simulink library "gyroscopes"  (R2023b)
settings: Solver=VariableStepAuto  StartTime=0.0  StopTime=10.0  RelTol=1e-3
undefined symbols (not defined in the file): gyr_bias, gyr_dynamic, gyr_freq, gyr_noise, gyr_non_orthogonality
libraries: simulink x1
settings Model: Creator=robin  LastModifiedBy=robin

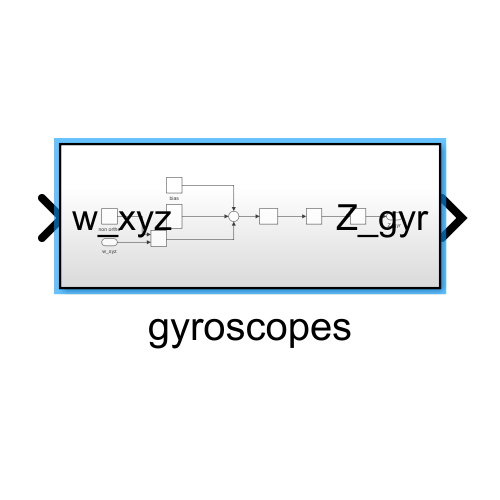
[thumbnail: Simulink's stored preview of the top-level diagram]
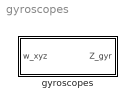
== system gyroscopes ==
  gyroscopes : Subsystem

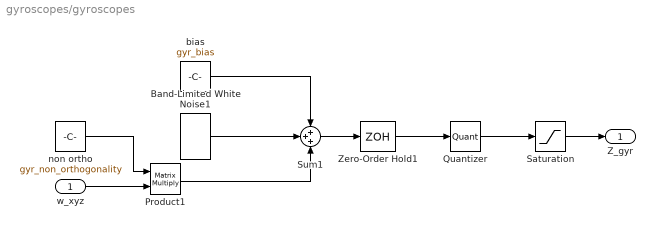
== system gyroscopes/gyroscopes ==
  w_xyz : Inport
  Band-Limited White Noise1 : simulink/Sources/Band-Limited White Noise  Cov=[2*(2*pi*gyr_noise/gyr_freq)^2 2*(2*pi*gyr_noise/gyr_freq)^2 2*(2*pi*gyr_noise/gyr_freq)^2]  Ts=1/gyr_freq  seed=[randi(1000) randi(1000) randi(1000)]  VectorParams1D=off
  Product1 : Product  Multiplication=Matrix(*)
  Quantizer : Quantizer  QuantizationInterval=gyr_res
  Saturation : Saturate  UpperLimit=gyr_dynamic  LowerLimit=-gyr_dynamic
  Sum1 : Sum  Inputs=+++
  Zero-Order Hold1 : ZeroOrderHold  SampleTime=1/gyr_freq
  bias : Constant  Value=gyr_bias
  non ortho : Constant  Value=gyr_non_orthogonality
  Z_gyr : Outport
  wires:
  non ortho/1 -> Product1/1
  Band-Limited White Noise1/1 -> Sum1/2
  bias/1 -> Sum1/1
  w_xyz/1 -> Product1/2
  Product1/1 -> Sum1/3
  Saturation/1 -> Z_gyr/1
  Zero-Order Hold1/1 -> Quantizer/1
  Sum1/1 -> Zero-Order Hold1/1
  Quantizer/1 -> Saturation/1
